simulink model "sample_rate2"  (Simulink 6.2)
settings: Solver=FixedStepDiscrete  StartTime=0.0  StopTime=1  RelTol=1e-3
libraries: dspsigops x2
settings Model: Creator=svenhoffmann  LastModifiedBy=svenhoffmann  ExtModeAutoUpdateStatusClock=off
settings DebuggingCC: SolverPrmCheckMsg=warning

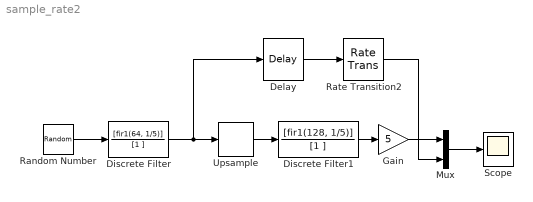
== system sample_rate2 ==
  Delay : dspsigops/Delay  dly_unit=Samples  delay=12  ic_detail=off  dif_ic_for_ch=off  dif_ic_for_dly=off  ic=0  reset_popup=None
  Discrete Filter : DiscreteFilter  Numerator=[fir1(64, 1/5)]  Denominator=[1 ]  SampleTime=-1
  Discrete Filter1 : DiscreteFilter  Numerator=[fir1(128, 1/5)]  Denominator=[1 ]  SampleTime=-1
  Gain : Gain  Gain=5
  Mux : Mux  Inputs=2
  Random Number : RandomNumber  SampleTime=1/1000
  Rate Transition2 : RateTransition
  Scope : Scope
  Upsample : dspsigops/Upsample  N=5  phase=0  ic=0  mode=Maintain input frame size
  wires:
  Random Number/1 -> Discrete Filter/1
  Discrete Filter/1 -> Upsample/1, Delay/1
  Upsample/1 -> Discrete Filter1/1
  Discrete Filter1/1 -> Gain/1
  Mux/1 -> Scope/1
  Gain/1 -> Mux/1
  Delay/1 -> Rate Transition2/1
  Rate Transition2/1 -> Mux/2
